simulink library "nmc"  (R2015b)
settings: Solver=ode45  SolverMode=SingleTasking  StartTime=0.0  StopTime=10.0  RelTol=1e-3
undefined symbols (not defined in the file): AnkleStance, AnkleSwing, c, c_jointstop, CtrlPar_FP_List, CtrlPar_FP_R_List, CtrlPar_LL_List, CtrlPar_St_List, CtrlPar_St_R_List, CtrlPar_Sw_List, CtrlPar_Sw_R_List, CtrlPar_theta0_List, CtrlPar_Tr_List, CtrlPar_Tr_R_List, CtrlPar_VelocityFile_List, D1G_HAT, eref, FmaxBFSH, FmaxGAS, FmaxGLU, FmaxHAB, FmaxHAD, FmaxHAM, FmaxHFL, FmaxRF, FmaxSOL, FmaxTA, FmaxVAS, init_a_tgt, init_a_tgtR, K, leg_l, LongDelay, LongLoopDelay, loptBFSH, loptGAS, loptGLU, loptHAB, loptHAD, loptHAM, loptHFL, loptRF, loptSOL, loptTA, loptVAS, lslackBFSH, lslackGAS, lslackGLU, lslackHAB, lslackHAD, lslackHAM, lslackHFL, lslackRF, lslackSOL, lslackTA, lslackVAS, magnitude, maxLoad_control_List, MeanStepsAnkle, MidDelay ... (+99)
libraries: nmc x63, simulink x31, simulink_extras x30, LopesDevelopmentLibrary x3
(part 2 of 10)

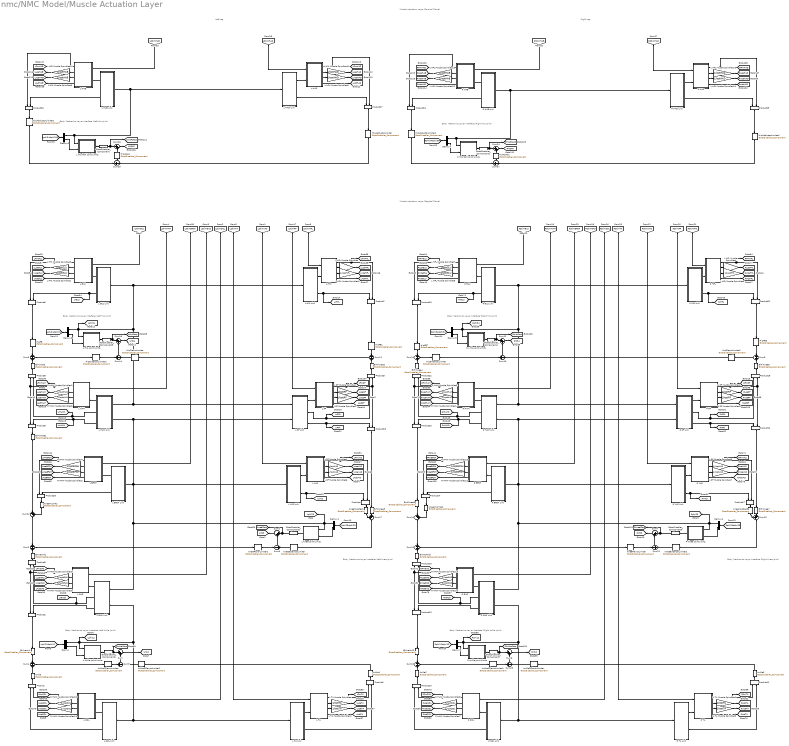
== system nmc/NMC Model/Muscle Actuation Layer ==
  note: Muscle Actuation Layer
      | (Coronal Plane)
  note: Right Leg
  note: Body Mechanics Layer
      | Interface (Right Hip Joint)
  note: Body Mechanics Layer
      | Interface (Left Hip Joint)
  note: Left Leg
  note: Body Mechanics Layer
      | Interface (Right Ankle Joint)
  note: Body Mechanics Layer
      | Interface (Right Knee Joint)
  note: Body Mechanics Layer
      | Interface (Right Hip Joint)
  note: Body Mechanics Layer
      | Interface (Left Ankle Joint)
  note: Body Mechanics Layer
      | Interface (Left Knee Joint)
  note: Body Mechanics Layer
      | Interface (Left Hip Joint)
  note: Muscle Actuation Layer
      | (Sagittal Plane)
  Ankle{,1..3} (4 alike) : nmc/GotoDisabler_Component  GotoTag=NMC_AnkleMuscles_Percentage
  AnkleDFlexorLimiter : nmc/GotoDisabler_Component  GotoTag=NMC_AnkleDFlexor_Percentage
  AnkleDFlexorLimiter1 : nmc/GotoDisabler_Component  GotoTag=NMC_AnkleDFlexor_Percentage
  AnklePFlexorLimiter : nmc/GotoDisabler_Component  GotoTag=NMC_AnklePFlexor_Percentage
  AnklePFlexorLimiter1 : nmc/GotoDisabler_Component  GotoTag=NMC_AnklePFlexor_Percentage
  BiHiKnee{,1..7} (8 alike) : nmc/GotoDisabler_Component  GotoTag=NMC_BiArticularMuscles_HK_Percentage
  BiKneAnk{,1..3} (4 alike) : nmc/GotoDisabler_Component  GotoTag=NMC_BiArticularMuscles_KA_Percentage
  Demux{,1..7} (8 alike) : Demux  Outputs=2
  GotoDisabler_Component{,1..7} (8 alike) : nmc/GotoDisabler_Component  GotoTag=DisableNMC_JointLimits
  HipAbAd : nmc/GotoDisabler_Component  GotoTag=NMC_HipAbAdMuscles_Percentage
  HipAbAd1 : nmc/GotoDisabler_Component  GotoTag=NMC_HipAbAdMuscles_Percentage
  HipAbductorLimiter1 : nmc/GotoDisabler_Component  GotoTag=NMC_HipAbductor_Percentage
  HipAbductorLimiter2 : nmc/GotoDisabler_Component  GotoTag=NMC_HipAbductor_Percentage
  HipAdductorLimiter : nmc/GotoDisabler_Component  GotoTag=NMC_HipAdductor_Percentage
  HipAdductorLimiter1 : nmc/GotoDisabler_Component  GotoTag=NMC_HipAdductor_Percentage
  HipExtensorLimiter : nmc/GotoDisabler_Component  GotoTag=NMC_HipExtensor_Percentage
  HipExtensorLimiter1 : nmc/GotoDisabler_Component  GotoTag=NMC_HipExtensor_Percentage
  HipFE{,1..3} (4 alike) : nmc/GotoDisabler_Component  GotoTag=NMC_HipFEMuscles_Percentage
  HipFlexorLimiter : nmc/GotoDisabler_Component  GotoTag=NMC_HipFlexor_Percentage
  HipFlexorLimiter1 : nmc/GotoDisabler_Component  GotoTag=NMC_HipFlexor_Percentage
  KneeExtensorLimiter : nmc/GotoDisabler_Component  GotoTag=NMC_KneeExtensor_Percentage
  KneeExtensorLimiter1 : nmc/GotoDisabler_Component  GotoTag=NMC_KneeExtensor_Percentage
  KneeFlexorLimiter : nmc/GotoDisabler_Component  GotoTag=NMC_KneeFlexor_Percentage
  KneeFlexorLimiter1 : nmc/GotoDisabler_Component  GotoTag=NMC_KneeFlexor_Percentage
  KneeMuscles{,1..3} (4 alike) : nmc/GotoDisabler_Component  GotoTag=NMC_KneeMuscles_Percentage
  L Ankle Joint Limits : Subsystem
  L BFSH : Subsystem
  L BFSH Link : Subsystem
  L GAS : Subsystem
  L GAS Link : Subsystem
  L GLU : Subsystem
  L GLU Link : Subsystem
  L HAB : Subsystem
  L HAB Link : Subsystem
  L HAD : Subsystem
  L HAD Link : Subsystem
  L HAM : Subsystem
  L HAM Link : Subsystem
  L HFL : Subsystem
  L HFL Muscle Spindles{,1,4..5} (4 alike) : Gain  Gain=1/loptHFL
  L HFL Muscle Spindles{9..10,12..13} (4 alike) : Gain  Gain=1/loptHAB
  L HFL Muscle Spindles{8,11,14..15} (4 alike) : Gain  Gain=1/loptHAD
  L HFL Muscle Spindles{2..3,6..7} (4 alike) : Gain  Gain=1/loptGLU
  L HFL Link : Subsystem
  L Hip Joint Limits : Subsystem
  L Hip Roll Joint Limits : Subsystem
  L Knee Joint Limits : Subsystem
  L RF : Subsystem
  L RF Muscle Spindles{,1..3} (4 alike) : Gain  Gain=1/loptRF
  L RF Muscle Spindles{4..7} (4 alike) : Gain  Gain=1/loptVAS
  L RF Link : Subsystem
  L SOL : Subsystem
  L SOL Link : Subsystem
  L TA : Subsystem
  L TA Muscle Spindles{,1..3} (4 alike) : Gain  Gain=1/loptTA
  L TA Link : Subsystem
  L VAS : Subsystem
  L VAS Link : Subsystem
  Product{,1..27} (28 alike) : Product  RndMeth=Zero
  R Ankle Joint Limits : Subsystem
  R BFSH : Subsystem
  R BFSH Link : Subsystem
  R GAS : Subsystem
  R GAS Link : Subsystem
  R GLU : Subsystem
  R GLU Link : Subsystem
  R HAB : Subsystem
  R HAB Link : Subsystem
  R HAD : Subsystem
  R HAD Link : Subsystem
  R HAM : Subsystem
  R HAM Muscle Spindles{1,3,6,14} (4 alike) : Gain  Gain=1/loptHAM
  R HAM Muscle Spindles{5,7,10..11} (4 alike) : Gain  Gain=1/loptSOL
  R HAM Muscle Spindles{2,4,12..13} (4 alike) : Gain  Gain=1/loptBFSH
  R HAM Muscle Spindles{8..9,15..16} (4 alike) : Gain  Gain=1/loptGAS
  R HAM Link : Subsystem
  R HFL : Subsystem
  R HFL Link : Subsystem
  R Hip Roll Joint Limits : Subsystem
  R Knee Joint Limits : Subsystem
  R L Hip Joint Limits : Subsystem
  R RF : Subsystem
  R RF Link : Subsystem
  R SOL : Subsystem
  R SOL Link : Subsystem
  R TA : Subsystem
  R TA Link : Subsystem
  R VAS : Subsystem
  R VAS Link : Subsystem
  Sum{,1,6..7,12,16,18,22,24,26} (10 alike) : Sum  Inputs=|++
  Sum{9..10,14,23,25,27} (6 alike) : Sum  Inputs=+-
  Sum{2..4,8,11,15,19..20} (8 alike) : Sum
  Sum13 : Sum  Inputs=++|
  Sum17 : Sum  Inputs=++|
  Sum21 : Sum  Inputs=-+
  Sum5 : Sum  Inputs=-+
  tag scope: LActBFSH=global, LActGAS=global, LActGLU=global, LActHAB=global, LActHAD=global, LActHAM=global, LActHFL=global, LActRF=global, LActSOL=global, LActTA=global, LActVAS=global, LAnkleStop=global, LFmBFSH=global, LFmGAS=global, LFmGLU=global, LFmHAB=global, LFmHAD=global, LFmHAM=global, LFmHFL=global, LFmRF=global, LFmSOL=global, LFmTA=global, LFmVAS=global, LHipRStop=global, LHipStop=global, LKneeStop=global, LLceBFSH=global, LLceGAS=global, LLceGLU=global, LLceHAB=global, LLceHAD=global, LLceHAM=global, LLceHFL=global, LLceRF=global, LLceSOL=global, LLceTA=global, LLceVAS=global, LM12=global, LM23=global, LM34=global, LM34R=global, LVceBFSH=global, LVceGAS=global, LVceGLU=global, LVceHAB=global, LVceHAD=global, LVceHAM=global, LVceHFL=global, LVceRF=global, LVceSOL=global, LVceTA=global, LVceVAS=global, Lphi12=global, Lphi23=global, Lphi34=global, LrGASk=global, LrGLU=global, LrHAMh=global, LrHAMk=global, LrHFL=global, LrRFh=global, LrRFk=global, LrVAS=global, RActBFSH=global, RActGAS=global, RActGLU=global, RActHAB=global, RActHAD=global, RActHAM=global, RActHFL=global, RActRF=global, RActSOL=global, RActTA=global, RActVAS=global, RAnkleStop=global, RFmBFSH=global, RFmGAS=global, RFmGLU=global, RFmHAB=global, RFmHAD=global, RFmHAM=global, RFmHFL=global, RFmRF=global, RFmSOL=global, RFmTA=global, RFmVAS=global, RHipStop=global, RHipStopR=global, RKneeStop=global, RLceBFSH=global, RLceGAS=global, RLceGLU=global, RLceHAB=global, RLceHAD=global, RLceHAM=global, RLceHFL=global, RLceRF=global, RLceSOL=global, RLceTA=global, RLceVAS=global, RM12=global, RM23=global, RM34=global, RM34R=global, RVceBFSH=global, RVceGAS=global, RVceGLU=global, RVceHAB=global, RVceHAD=global, RVceHAM=global, RVceHFL=global, RVceRF=global, RVceSOL=global, RVceTA=global, RVceVAS=global, Rphi12=global, Rphi23=global, Rphi34=global, RrGASk=global, RrGLU=global, RrHAMh=global, RrHAMk=global, RrHFL=global, RrRFh=global, RrRFk=global, RrVAS=global
  wires:
  L HFL/1(Fmtc) -> [LFmHFL], Product7/2
  [LStimHFL] -> L HFL/1(STIM)
  Product7/1 -> HipFE1/1
  Ankle3/1 -> AnkleDFlexorLimiter/1
  Ankle2/1 -> Sum20/2
  Ankle1/1 -> AnkleDFlexorLimiter1/1
  Ankle/1 -> Sum4/2
  BiKneAnk3/1 -> Sum15/2
  Product16/1 -> BiKneAnk3/1
  BiKneAnk2/1 -> Sum20/1
  BiKneAnk1/1 -> Sum2/2
  Product3/1 -> BiKneAnk1/1
  BiKneAnk/1 -> Sum4/1
  KneeMuscles3/1 -> Sum13/1
  KneeMuscles2/1 -> Sum18/2
  KneeMuscles1/1 -> Sum17/1
  KneeMuscles/1 -> Sum22/2
  Sum22/1 -> Sum2/1
  BiHiKnee7/1 -> Sum13/2
  BiHiKnee6/1 -> Sum8/2
  BiHiKnee5/1 -> Sum18/1
  BiHiKnee4/1 -> Sum19/2
  BiHiKnee3/1 -> Sum17/2
  BiHiKnee2/1 -> Sum11/2
  BiHiKnee1/1 -> Sum22/1
  Product8/1 -> BiHiKnee/1
  BiHiKnee/1 -> Sum3/2
  HipFE3/1 -> Sum8/1
  HipFE2/1 -> Sum19/1
  HipFE1/1 -> Sum11/1
  HipFE/1 -> Sum3/1
  HipAbAd1/1 -> Sum24/2
  Sum27/1 -> HipAbAd1/1
  HipAbAd/1 -> Sum26/2
  Sum25/1 -> HipAbAd/1
  AnkleDFlexorLimiter/1 -> Sum23/2
  AnkleDFlexorLimiter1/1 -> Sum9/2
  HipFlexorLimiter1/1 -> Sum10/2
  HipExtensorLimiter/1 -> Sum10/1
  HipFlexorLimiter/1 -> Sum14/2
  HipExtensorLimiter1/1 -> Sum14/1
  AnklePFlexorLimiter/1 -> Sum9/1
  AnklePFlexorLimiter1/1 -> Sum23/1
  KneeExtensorLimiter1/1 -> Sum21/2
  KneeFlexorLimiter/1 -> Sum21/1
  KneeExtensorLimiter/1 -> Sum5/2
  KneeFlexorLimiter1/1 -> Sum5/1
  Product9/1 -> BiHiKnee1/1
  HipAdductorLimiter1/1 -> Sum27/2
  HipAdductorLimiter/1 -> Sum25/2
  HipAbductorLimiter1/1 -> Sum27/1
  HipAbductorLimiter2/1 -> Sum25/1
  Product1/1 -> Ankle1/1
  Product11/1 -> Ankle3/1
  Product10/1 -> Ankle2/1
  Product/1 -> Ankle/1
  Product6/1 -> HipFE/1
  Product19/1 -> HipFE2/1
  Product21/1 -> HipFE3/1
  Product20/1 -> KneeMuscles/1
  Product14/1 -> KneeMuscles2/1
  Product17/1 -> KneeMuscles3/1
  Product4/1 -> KneeMuscles1/1
  R Ankle Joint Limits/1(M_stop [Nm]) -> GotoDisabler_Component7/1
  GotoDisabler_Component5/1 -> [LHipStop], Sum16/1
  L Hip Joint Limits/1(M_stop [Nm]) -> GotoDisabler_Component5/1
  GotoDisabler_Component4/1 -> Sum12/1, [RHipStop]
  R L Hip Joint Limits/1(M_stop [Nm]) -> GotoDisabler_Component4/1
  GotoDisabler_Component1/1 -> [RHipStopR], Sum24/1
  GotoDisabler_Component/1 -> [LHipRStop], Sum26/1
  GotoDisabler_Component2/1 -> [LKneeStop], Sum1/1
  GotoDisabler_Component3/1 -> [RKneeStop], Sum7/1
  GotoDisabler_Component6/1 -> [LAnkleStop], Sum/1
  GotoDisabler_Component7/1 -> [RAnkleStop], Sum6/1
  Sum/1 -> [LM12]
  R HAD/1(Fmtc) -> Product25/2, [RFmHAD]
  R HAD/4(A) -> [RActHAD]
  R HAD/3(Vce) -> L HFL Muscle Spindles14/1
  R HAD/2(Lce) -> L HFL Muscle Spindles15/1
  L HFL Muscle Spindles15/1 -> [RLceHAD]
  L HFL Muscle Spindles14/1 -> [RVceHAD]
  R HAB/1(Fmtc) -> Product24/1, [RFmHAB]
  L HFL Muscle Spindles13/1 -> [RLceHAB]
  L HFL Muscle Spindles12/1 -> [RVceHAB]
  R HAB/3(Vce) -> L HFL Muscle Spindles12/1
  R HAB/2(Lce) -> L HFL Muscle Spindles13/1
  R HAB/4(A) -> [RActHAB]
  L HAD/1(Fmtc) -> Product27/2, [LFmHAD]
  L HAD/4(A) -> [LActHAD]
  L HAD/3(Vce) -> L HFL Muscle Spindles8/1
  L HAD/2(Lce) -> L HFL Muscle Spindles11/1
  L HFL Muscle Spindles11/1 -> [LLceHAD]
  L HFL Muscle Spindles8/1 -> [LVceHAD]
  L HAB/1(Fmtc) -> [LFmHAB], Product26/1
  L HFL Muscle Spindles10/1 -> [LLceHAB]
  L HFL Muscle Spindles9/1 -> [LVceHAB]
  L HAB/3(Vce) -> L HFL Muscle Spindles9/1
  L HAB/2(Lce) -> L HFL Muscle Spindles10/1
  L HAB/4(A) -> [LActHAB]
  [RStimHAB] -> R HAB/1(STIM)
  R HAD Link/2(lever [m]) -> Product25/1
  R HAD Link/1(lmtu [m]) -> R HAD/2(lmtc [m])
  Product25/1 -> HipAdductorLimiter1/1
  R Hip Roll Joint Limits/1(M_stop [Nm]) -> GotoDisabler_Component1/1
  Demux7/2 -> R Hip Roll Joint Limits/2(dphi [rad/s])
  R HAB Link/2(lever [m]) -> Product24/2
  R HAB Link/1(lmtu [m]) -> R HAB/2(lmtc [m])
  Product24/1 -> HipAbductorLimiter1/1
  Demux7/1 -> R Hip Roll Joint Limits/1(phi [rad]), R HAB Link/1(phi34R [rad]), R HAD Link/1(phi34R [rad])
  [Rphi34dphi34R] -> Demux7/1
  Sum24/1 -> [RM34R]
  [RStimHAD] -> R HAD/1(STIM)
  L HAD Link/2(lever [m]) -> Product27/1
  L HAD Link/1(lmtu [m]) -> L HAD/2(lmtc [m])
  Product27/1 -> HipAdductorLimiter/1
  L Hip Roll Joint Limits/1(M_stop [Nm]) -> GotoDisabler_Component/1
  Demux6/2 -> L Hip Roll Joint Limits/2(dphi [rad/s])
  L HAB Link/2(lever [m]) -> Product26/2
  L HAB Link/1(lmtu [m]) -> L HAB/2(lmtc [m])
  Product26/1 -> HipAbductorLimiter2/1
  Demux6/1 -> L Hip Roll Joint Limits/1(phi [rad]), L HAD Link/1(phi34R [rad]), L HAB Link/1(phi34R [rad])
  [Lphi34dphi34R] -> Demux6/1
  Sum26/1 -> [LM34R]
  [LStimHAB] -> L HAB/1(STIM)
  [LStimHAD] -> L HAD/1(STIM)
  Sum11/1 -> HipFlexorLimiter/1
  L TA Muscle Spindles2/1 -> [RLceTA]
  L RF Muscle Spindles5/1 -> [RLceVAS]
  R HAM Muscle Spindles12/1 -> [RVceBFSH]
  R HAM Muscle Spindles13/1 -> [RLceBFSH]
  L RF Muscle Spindles3/1 -> [RVceRF]
  L RF Muscle Spindles1/1 -> [RLceRF]
  R HAM Muscle Spindles14/1 -> [RVceHAM]
  R HAM Muscle Spindles3/1 -> [RLceHAM]
  L HFL Muscle Spindles4/1 -> [RLceHFL]
  L TA Muscle Spindles3/1 -> [RVceTA]
  R TA/1(Fmtc) -> [RFmTA], Product11/1
  R HAM Muscle Spindles7/1 -> [RVceSOL]
  R HAM Muscle Spindles5/1 -> [RLceSOL]
  R HAM Muscle Spindles16/1 -> [RVceGAS]
  R HAM Muscle Spindles15/1 -> [RLceGAS]
  R BFSH/1(Fmtc) -> [RFmBFSH], Product14/1
  R RF/1(Fmtc) -> [RFmRF], Product12/2, Product18/2
  L RF Muscle Spindles7/1 -> [RVceVAS]
  L HFL Muscle Spindles7/1 -> [RLceGLU]
  L HFL Muscle Spindles6/1 -> [RVceGLU]
  L HFL Muscle Spindles5/1 -> [RVceHFL]
  Product23/1 -> BiHiKnee5/1
  Sum18/1 -> Sum15/1
  R BFSH/3(Vce) -> R HAM Muscle Spindles12/1
  R BFSH/2(Lce) -> R HAM Muscle Spindles13/1
  R BFSH/4(A) -> [RActBFSH]
  R BFSH Link/2(lever [m]) -> Product14/2
  R BFSH Link/1(lmtu [m]) -> R BFSH/2(lmtc [m])
  [RStimBFSH] -> R BFSH/1(STIM)
  Sum13/1 -> KneeExtensorLimiter1/1
  Product12/1 -> BiHiKnee7/1
  Product18/1 -> BiHiKnee6/1
  Sum8/1 -> HipFlexorLimiter1/1
  [RStimRF] -> R RF/1(STIM)
  R RF Link/3(lever23 [m]) -> [RrRFk], Product12/1
  R RF Link/2(lever34 [m]) -> [RrRFh], Product18/1
  R RF Link/1(lmtu [m]) -> R RF/2(lmtc [m])
  R RF/2(Lce) -> L RF Muscle Spindles1/1
  R RF/3(Vce) -> L RF Muscle Spindles3/1
  R RF/4(A) -> [RActRF]
  R HFL/3(Vce) -> L HFL Muscle Spindles5/1
  R VAS/2(Lce) -> L RF Muscle Spindles5/1
  R VAS/3(Vce) -> L RF Muscle Spindles7/1
  R TA/3(Vce) -> L TA Muscle Spindles3/1
  R SOL/3(Vce) -> R HAM Muscle Spindles7/1
  R SOL/2(Lce) -> R HAM Muscle Spindles5/1
  R GAS/2(Lce) -> R HAM Muscle Spindles15/1
  R GAS/3(Vce) -> R HAM Muscle Spindles16/1
  R HAM/3(Vce) -> R HAM Muscle Spindles14/1
  R GLU/3(Vce) -> L HFL Muscle Spindles6/1
  R GLU/2(Lce) -> L HFL Muscle Spindles7/1
  [RStimVAS] -> R VAS/1(STIM)
  R HFL Link/2(lever [m]) -> [RrHFL], Product21/1
  R HFL/4(A) -> [RActHFL]
  R HFL Link/1(lmtu [m]) -> R HFL/2(lmtc [m])
  Sum10/1 -> Sum12/2
  Demux5/2 -> R L Hip Joint Limits/2(dphi [rad/s])
  R GLU/4(A) -> [RActGLU]
  R GLU Link/2(lever [m]) -> [RrGLU], Product19/2
  R GLU Link/1(lmtu [m]) -> R GLU/2(lmtc [m])
  Product22/1 -> BiHiKnee4/1
  R HAM/4(A) -> [RActHAM]
  Sum15/1 -> KneeFlexorLimiter/1
  R VAS Link/2(lever [m]) -> Product17/1, [RrVAS]
  Sum21/1 -> Sum7/2
  R Knee Joint Limits/1(M_stop [Nm]) -> GotoDisabler_Component3/1
  Sum7/1 -> [RM23]
  R VAS/1(Fmtc) -> [RFmVAS], Product17/2
  R VAS/4(A) -> [RActVAS]
  R GAS/4(A) -> [RActGAS]
  R SOL/4(A) -> [RActSOL]
  Sum6/1 -> [RM12]
  R TA Link/2(lever [m]) -> Product11/2
  Product13/1 -> BiKneAnk2/1
  R SOL Link/2(lever [m]) -> Product10/1
  Demux5/1 -> [Rphi34], R HAM Link/1(phi34 [rad]), R RF Link/1(phi34 [rad]), R GLU Link/1(phi34 [rad]), R HFL Link/1(phi34 [rad]), R L Hip Joint Limits/1(phi [rad])
  [Rphi34dphi34] -> Demux5/1
  [Rphi23dphi23] -> Demux4/1
  [Rphi12dphi12] -> Demux3/1
  Sum20/1 -> AnklePFlexorLimiter1/1
  Sum19/1 -> HipExtensorLimiter/1
  R HAM Link/3(lever23 [m]) -> [RrHAMk], Product23/2
  R HAM Link/2(lever34 [m]) -> [RrHAMh], Product22/2
  R HAM Link/1(lmtu [m]) -> R HAM/2(lmtc [m])
  R VAS Link/1(lmtu [m]) -> R VAS/2(lmtc [m])
  R GAS Link/1(lmtu [m]) -> R GAS/2(lmtc [m])
  [RStimGAS] -> R GAS/1(STIM)
  R GAS Link/2(lever23 [m]) -> [RrGASk], Product16/2
  R GAS Link/3(lever12 [m]) -> Product13/2
  R TA Link/1(lmtc [m]) -> R TA/2(lmtc [m])
  R SOL Link/1(lmtc [m]) -> R SOL/2(lmtc [m])
  Demux4/2 -> R Knee Joint Limits/2(dphi [rad/s])
  Sum23/1 -> Sum6/2
  Demux3/2 -> R Ankle Joint Limits/2(dphi [rad/s])
  Sum12/1 -> [RM34]
  [RStimGLU] -> R GLU/1(STIM)
  R GLU/1(Fmtc) -> [RFmGLU], Product19/1
  [RStimHFL] -> R HFL/1(STIM)
  R HFL/2(Lce) -> L HFL Muscle Spindles4/1
  R HFL/1(Fmtc) -> [RFmHFL], Product21/2
  R HAM/2(Lce) -> R HAM Muscle Spindles3/1
  R HAM/1(Fmtc) -> [RFmHAM], Product22/1, Product23/1
  [RStimHAM] -> R HAM/1(STIM)
  [RStimSOL] -> R SOL/1(STIM)
  [RStimTA] -> R TA/1(STIM)
  Demux3/1 -> [Rphi12], R Ankle Joint Limits/1(phi [rad]), R GAS Link/2(phi12 [rad]), R TA Link/1(phi12 [rad]), R SOL Link/1(phi12 [rad])
  R GAS/1(Fmtc) -> [RFmGAS], Product16/1, Product13/1
  R TA/4(A) -> [RActTA]
  R TA/2(Lce) -> L TA Muscle Spindles2/1
  R SOL/1(Fmtc) -> [RFmSOL], Product10/2
  Demux4/1 -> [Rphi23], R GAS Link/1(phi23 [rad]), R BFSH Link/1(phi23 [rad]), R HAM Link/2(phi23 [rad]), R RF Link/2(phi23 [rad]), R VAS Link/1(phi23 [rad]), R Knee Joint Limits/1(phi [rad])
  L TA Muscle Spindles/1 -> [LLceTA]
  L RF Muscle Spindles4/1 -> [LLceVAS]
  R HAM Muscle Spindles2/1 -> [LVceBFSH]
  R HAM Muscle Spindles4/1 -> [LLceBFSH]
  L RF Muscle Spindles2/1 -> [LVceRF]
  L RF Muscle Spindles/1 -> [LLceRF]
  R HAM Muscle Spindles6/1 -> [LVceHAM]
  R HAM Muscle Spindles1/1 -> [LLceHAM]
  L HFL Muscle Spindles/1 -> [LLceHFL]
  L TA Muscle Spindles1/1 -> [LVceTA]
  L TA/1(Fmtc) -> [LFmTA], Product1/1
  R HAM Muscle Spindles11/1 -> [LVceSOL]
  R HAM Muscle Spindles10/1 -> [LLceSOL]
  R HAM Muscle Spindles9/1 -> [LVceGAS]
  R HAM Muscle Spindles8/1 -> [LLceGAS]
  L BFSH/1(Fmtc) -> [LFmBFSH], Product20/1
  L RF/1(Fmtc) -> [LFmRF], Product15/2, Product5/2
  L RF Muscle Spindles6/1 -> [LVceVAS]
  L HFL Muscle Spindles3/1 -> [LLceGLU]
  L HFL Muscle Spindles2/1 -> [LVceGLU]
  L HFL Muscle Spindles1/1 -> [LVceHFL]
  L BFSH/3(Vce) -> R HAM Muscle Spindles2/1
  L BFSH/2(Lce) -> R HAM Muscle Spindles4/1
  L BFSH/4(A) -> [LActBFSH]
  L BFSH Link/2(lever [m]) -> Product20/2
  L BFSH Link/1(lmtu [m]) -> L BFSH/2(lmtc [m])
  [LStimBFSH] -> L BFSH/1(STIM)
  Sum17/1 -> KneeExtensorLimiter/1
  Product15/1 -> BiHiKnee3/1
  Product5/1 -> BiHiKnee2/1
  [LStimRF] -> L RF/1(STIM)
  L RF Link/3(lever23 [m]) -> [LrRFk], Product15/1
  L RF Link/2(lever34 [m]) -> [LrRFh], Product5/1
  L RF Link/1(lmtu [m]) -> L RF/2(lmtc [m])
  L RF/2(Lce) -> L RF Muscle Spindles/1
  L RF/3(Vce) -> L RF Muscle Spindles2/1
  L RF/4(A) -> [LActRF]
  L HFL/3(Vce) -> L HFL Muscle Spindles1/1
  L VAS/2(Lce) -> L RF Muscle Spindles4/1
  L VAS/3(Vce) -> L RF Muscle Spindles6/1
  L TA/3(Vce) -> L TA Muscle Spindles1/1
  L SOL/3(Vce) -> R HAM Muscle Spindles11/1
  L SOL/2(Lce) -> R HAM Muscle Spindles10/1
  L GAS/2(Lce) -> R HAM Muscle Spindles8/1
  L GAS/3(Vce) -> R HAM Muscle Spindles9/1
  L HAM/3(Vce) -> R HAM Muscle Spindles6/1
  L GLU/3(Vce) -> L HFL Muscle Spindles2/1
  L GLU/2(Lce) -> L HFL Muscle Spindles3/1
  [LStimVAS] -> L VAS/1(STIM)
  L HFL Link/2(lever [m]) -> [LrHFL], Product7/1
  L HFL/4(A) -> [LActHFL]
  L HFL Link/1(lmtu [m]) -> L HFL/2(lmtc [m])
  Sum14/1 -> Sum16/2
  Demux2/2 -> L Hip Joint Limits/2(dphi [rad/s])
  L GLU/4(A) -> [LActGLU]
  L GLU Link/2(lever [m]) -> [LrGLU], Product6/2
  L GLU Link/1(lmtu [m]) -> L GLU/2(lmtc [m])
  L HAM/4(A) -> [LActHAM]
  Sum2/1 -> KneeFlexorLimiter1/1
  L VAS Link/2(lever [m]) -> Product4/1, [LrVAS]
  Sum5/1 -> Sum1/2
  L Knee Joint Limits/1(M_stop [Nm]) -> GotoDisabler_Component2/1
  Sum1/1 -> [LM23]
  L VAS/1(Fmtc) -> [LFmVAS], Product4/2
  L VAS/4(A) -> [LActVAS]
  L GAS/4(A) -> [LActGAS]
  L SOL/4(A) -> [LActSOL]
  L Ankle Joint Limits/1(M_stop [Nm]) -> GotoDisabler_Component6/1
  L TA Link/2(lever [m]) -> Product1/2
  Product2/1 -> BiKneAnk/1
  L SOL Link/2(lever [m]) -> Product/1
  Demux2/1 -> [Lphi34], L HAM Link/1(phi34 [rad]), L RF Link/1(phi34 [rad]), L GLU Link/1(phi34 [rad]), L HFL Link/1(phi34 [rad]), L Hip Joint Limits/1(phi [rad])
  [Lphi34dphi34] -> Demux2/1
  [Lphi23dphi23] -> Demux1/1
  [Lphi12dphi12] -> Demux/1
  Sum4/1 -> AnklePFlexorLimiter/1
  Sum3/1 -> HipExtensorLimiter1/1
  L HAM Link/3(lever23 [m]) -> [LrHAMk], Product9/2
  L HAM Link/2(lever34 [m]) -> [LrHAMh], Product8/2
  L HAM Link/1(lmtu [m]) -> L HAM/2(lmtc [m])
  L VAS Link/1(lmtu [m]) -> L VAS/2(lmtc [m])
  L GAS Link/1(lmtu [m]) -> L GAS/2(lmtc [m])
  [LStimGAS] -> L GAS/1(STIM)
  L GAS Link/2(lever23 [m]) -> [LrGASk], Product3/2
  L GAS Link/3(lever12 [m]) -> Product2/2
  L TA Link/1(lmtc [m]) -> L TA/2(lmtc [m])
  L SOL Link/1(lmtc [m]) -> L SOL/2(lmtc [m])
  Demux1/2 -> L Knee Joint Limits/2(dphi [rad/s])
  Sum9/1 -> Sum/2
  Demux/2 -> L Ankle Joint Limits/2(dphi [rad/s])
  Sum16/1 -> [LM34]
  [LStimGLU] -> L GLU/1(STIM)
  L GLU/1(Fmtc) -> [LFmGLU], Product6/1
  L HFL/2(Lce) -> L HFL Muscle Spindles/1
  L HAM/2(Lce) -> R HAM Muscle Spindles1/1
  L HAM/1(Fmtc) -> [LFmHAM], Product8/1, Product9/1
  [LStimHAM] -> L HAM/1(STIM)
  [LStimSOL] -> L SOL/1(STIM)
  [LStimTA] -> L TA/1(STIM)
  Demux/1 -> [Lphi12], L Ankle Joint Limits/1(phi [rad]), L GAS Link/2(phi12 [rad]), L TA Link/1(phi12 [rad]), L SOL Link/1(phi12 [rad])
  L GAS/1(Fmtc) -> [LFmGAS], Product3/1, Product2/1
  L TA/4(A) -> [LActTA]
  L TA/2(Lce) -> L TA Muscle Spindles/1
  L SOL/1(Fmtc) -> [LFmSOL], Product/2
  Demux1/1 -> [Lphi23], L GAS Link/1(phi23 [rad]), L BFSH Link/1(phi23 [rad]), L HAM Link/2(phi23 [rad]), L RF Link/2(phi23 [rad]), L VAS Link/1(phi23 [rad]), L Knee Joint Limits/1(phi [rad])

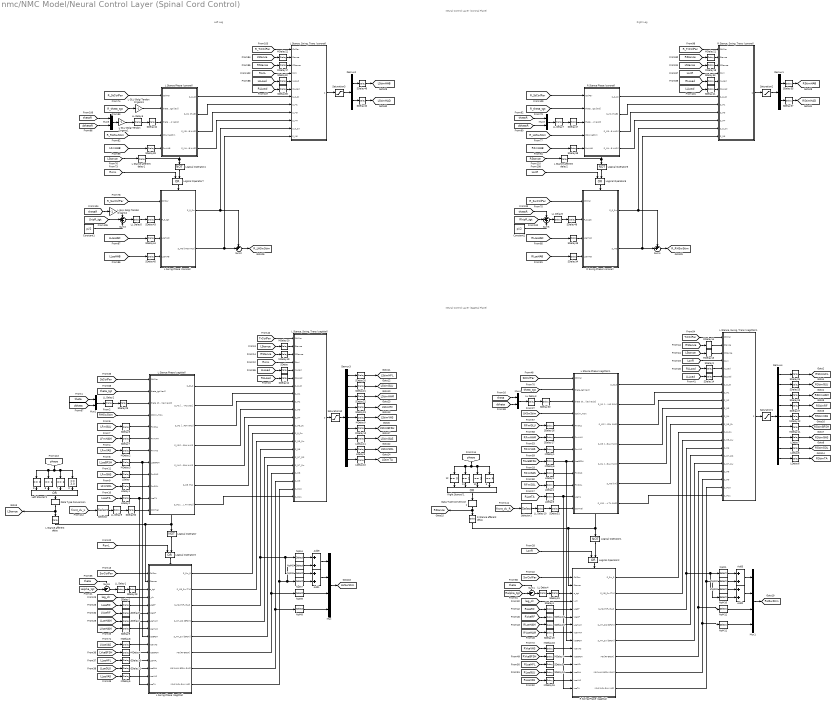
== system nmc/NMC Model/Neural Control Layer (Spinal Cord Control) ==
  note: Neural Control Layer
      | (Sagittal Plane)
  note: Neural Control Layer
      | (Coronal Plane)
  note: Right Leg
  note: Left Leg
  " 2" : simulink/Logic and Bit Operations/Compare To Constant  relop===  const=3.0  OutDataTypeStr=boolean
  " 3" : simulink/Logic and Bit Operations/Compare To Constant  relop===  const=4  OutDataTypeStr=boolean
  10 : simulink/Logic and Bit Operations/Compare To Constant  relop===  const=3  OutDataTypeStr=boolean
  11 : simulink/Logic and Bit Operations/Compare To Constant  relop===  const=1  OutDataTypeStr=boolean
  12 : simulink/Logic and Bit Operations/Compare To Constant  relop===  const=0  OutDataTypeStr=boolean
  7 : simulink/Logic and Bit Operations/Compare To Constant  relop===  const=2  OutDataTypeStr=boolean
  8 : simulink/Logic and Bit Operations/Compare To Constant  relop===  const=1  OutDataTypeStr=boolean
  9 : simulink/Logic and Bit Operations/Compare To Constant  relop===  const=0  OutDataTypeStr=boolean
  Add{1..3,9} (4 alike) : Sum  Inputs=2
  Constant1 : Constant  Value=pi/2
  Constant2 : Constant  Value=pi/2
  Data Type Conversion : DataTypeConversion
  Data Type Conversion1 : DataTypeConversion
  Demux1 : Demux  Outputs=2
  Demux2 : Demux  Outputs=2
  Demux3 : Demux  Outputs=9
  Demux4 : Demux  Outputs=9
  L GLU Golgi Tendon Organs1 : Gain  Gain=-1
  L GLU Golgi Tendon Organs2 : Gain  Gain=-1
  L GLU Golgi Tendon Organs3 : Gain  Gain=-1
  L Stance afferent delay : TransportDelay  DelayTime=MidDelay
  L Stance afferent delay1 : TransportDelay  DelayTime=MidDelay
  L Stance afferent delay2 : TransportDelay  DelayTime=MidDelay
  L Stance Phase (coronal) : Subsystem  TreatAsAtomicUnit=on
  L Stance Phase (sagittal) : Subsystem  TreatAsAtomicUnit=on
  L Stance Phase (sagittal)1 : Subsystem  TreatAsAtomicUnit=on
  "L Stance, Swing, Trans (coronal)" : Subsystem  TreatAsAtomicUnit=on
  "L Stance, Swing, Trans (sagittal)" : Subsystem
  "L Stance, Swing, Trans (sagittal)1" : Subsystem
  L Swing Phase (coronal) : Subsystem  TreatAsAtomicUnit=on
  L Swing Phase (sagittal) : Subsystem  TreatAsAtomicUnit=on
  LDelay{,1,3..4} (4 alike) : TransportDelay  DelayTime=LongDelay
  LDelay10 : TransportDelay  DelayTime=LongDelay  InitialOutput=St_PreSTA
  LDelay11 : TransportDelay  DelayTime=LongDelay  InitialOutput=St_PreSGAS
  LDelay2 : TransportDelay  DelayTime=LongDelay  InitialOutput=1
  LDelay5 : TransportDelay  DelayTime=LongDelay  InitialOutput=1
  LDelay6 : TransportDelay  DelayTime=LongDelay  InitialOutput=Sw_PreSTA
  LDelay7 : TransportDelay  DelayTime=LongDelay  InitialOutput=Sw_PreSGAS
  LDelay8 : TransportDelay  DelayTime=LongDelay  InitialOutput=Sw_PreSSOL
  LDelay9 : TransportDelay  DelayTime=LongDelay  InitialOutput=St_PreSSOL
  LL Delay1 : TransportDelay  DelayTime=LongLoopDelay/2  InitialOutput=init_a_tgt
  LL Delay{2..3,6..7,9..10} (6 alike) : TransportDelay  DelayTime=LongLoopDelay/2
  LL Delay4 : TransportDelay  DelayTime=LongLoopDelay/2  InitialOutput=init_a_tgt
  LL Delay5 : TransportDelay  DelayTime=LongLoopDelay/2  InitialOutput=init_a_tgtR
  LL Delay8 : TransportDelay  DelayTime=LongLoopDelay/2  InitialOutput=init_a_tgtR
  Left Stance?2 : Logic  Operator=OR  Inputs=4  AllPortsSameDT=off
  Logical Operator{,1,4..5} (4 alike) : Logic  Operator=NOT  AllPortsSameDT=off  OutDataTypeStr=boolean
  Logical Operator{2..3,6..7} (4 alike) : Logic  Operator=OR  AllPortsSameDT=off  OutDataTypeStr=boolean
  MDelay{1..2,4,7..8,13..14,16..22} (14 alike) : TransportDelay  DelayTime=MidDelay
  MDelay10 : TransportDelay  DelayTime=MidDelay  InitialOutput=St_PreSBFSH
  MDelay11 : TransportDelay  DelayTime=MidDelay  InitialOutput=Sw_PreSBFSH
  MDelay12 : TransportDelay  DelayTime=MidDelay  InitialOutput=Sw_PreSVAS
  MDelay{3,5..6,15} (4 alike) : TransportDelay  DelayTime=MidDelay  InitialOutput=1
  MDelay9 : TransportDelay  DelayTime=MidDelay  InitialOutput=St_PreSVAS
  Mux : Mux
  Mux1 : Mux
  Mux{2..5} (4 alike) : Mux  Inputs=2
  R Stance afferent delay : TransportDelay  DelayTime=MidDelay
  R Stance Phase (coronal) : Subsystem  TreatAsAtomicUnit=on
  "R Stance, Swing, Trans (coronal)" : Subsystem  TreatAsAtomicUnit=on
  R Swing Phase (coronal) : Subsystem  TreatAsAtomicUnit=on
  R Swing Phase (sagittal) : Subsystem  TreatAsAtomicUnit=on
  Right Stance?1 : Logic  Operator=OR  Inputs=4  AllPortsSameDT=off
  SDelay{,3,6..9,12,14,16..19,29..30,32..33,36,38..39,41..42,47,50..51} (24 alike) : TransportDelay  DelayTime=ShortDelay
  SDelay{1..2,4..5,10..11,13,15,34,44..45,49} (12 alike) : TransportDelay  DelayTime=ShortDelay  InitialOutput=1
  SDelay20 : TransportDelay  DelayTime=ShortDelay  InitialOutput=St_PreSHFL
  SDelay21 : TransportDelay  DelayTime=ShortDelay  InitialOutput=St_PreSGLU
  SDelay22 : TransportDelay  DelayTime=ShortDelay  InitialOutput=St_PreSHAM
  SDelay23 : TransportDelay  DelayTime=ShortDelay  InitialOutput=St_PreSRF
  SDelay24 : TransportDelay  DelayTime=ShortDelay  InitialOutput=Sw_PreSHFL
  SDelay25 : TransportDelay  DelayTime=ShortDelay  InitialOutput=Sw_PreSGLU
  SDelay26 : TransportDelay  DelayTime=ShortDelay  InitialOutput=Sw_PreSHAM
  SDelay27 : TransportDelay  DelayTime=ShortDelay  InitialOutput=Sw_PreSRF
  SDelay28 : TransportDelay  DelayTime=ShortDelay  InitialOutput=init_a_tgt
  SDelay31 : TransportDelay  DelayTime=ShortDelay  InitialOutput=init_a_tgt
  SDelay35 : TransportDelay  DelayTime=ShortDelay  InitialOutput=Sw_PreS_HAB
  SDelay37 : TransportDelay  DelayTime=ShortDelay  InitialOutput=Sw_PreS_HAD
  SDelay40 : TransportDelay  DelayTime=ShortDelay  InitialOutput=St_PreS_HAD
  SDelay43 : TransportDelay  DelayTime=ShortDelay  InitialOutput=init_a_tgtR
  SDelay46 : TransportDelay  DelayTime=ShortDelay  InitialOutput=St_PreS_HAB
  SDelay48 : TransportDelay  DelayTime=ShortDelay  InitialOutput=init_a_tgtR
  Saturation{1..3,10} (4 alike) : Saturate  UpperLimit=1  LowerLimit=0.01  ZeroCross=off
  Selector : Selector  InputPortWidth=2  IndexOptions=Index vector (dialog)  Indices=[2]  OutputSizes=1
  Selector1 : Selector  InputPortWidth=2  IndexOptions=Index vector (dialog)  Indices=[2]  OutputSizes=1
  Sum1 : Sum  Inputs=-+|
  Sum2 : Sum  Inputs=++|
  Sum3 : Sum  Inputs=--+
  Sum4 : Sum  Inputs=++|
  Sum5 : Sum  Inputs=--+
  Sum6 : Sum  Inputs=-+|
  hipM{1,4,9,12} (4 alike) : Selector  InputPortWidth=2  IndexOptions=Index vector (dialog)  Indices=1  OutputSizes=1
  hipM10 : Selector  InputPortWidth=3  IndexOptions=Index vector (dialog)  Indices=2  OutputSizes=1
  hipM{2,5,8,11} (4 alike) : Selector  InputPortWidth=3  IndexOptions=Index vector (dialog)  Indices=1  OutputSizes=1
  hipM3 : Selector  InputPortWidth=2  IndexOptions=Index vector (dialog)  Indices=2  OutputSizes=1
  hipM6 : Selector  InputPortWidth=2  IndexOptions=Index vector (dialog)  Indices=2  OutputSizes=1
  hipM7 : Selector  InputPortWidth=3  IndexOptions=Index vector (dialog)  Indices=2  OutputSizes=1
  tag scope: LHSwStim=global, LStance=global, LStimBFSH=global, LStimGAS=global, LStimGLU=global, LStimHAB=global, LStimHAD=global, LStimHAM=global, LStimHFL=global, LStimRF=global, LStimSOL=global, LStimTA=global, LStimVAS=global, RHSwStim=global, RStance=global, RStimBFSH=global, RStimGAS=global, RStimGLU=global, RStimHAB=global, RStimHAD=global, RStimHAM=global, RStimHFL=global, RStimRF=global, RStimSOL=global, RStimTA=global, RStimVAS=global, R_LHSwStim=global, R_RHSwStim=global
  wires:
  Data Type Conversion1/1 -> R Stance afferent delay/1, [RStance]
  Data Type Conversion/1 -> L Stance afferent delay/1, [LStance]
  [phase] -> 11/1, 12/1, 10/1, " 3"/1
  " 3"/1 -> Right Stance?1/4
  10/1 -> Right Stance?1/3
  11/1 -> Right Stance?1/2
  12/1 -> Right Stance?1/1
  [phase] -> 8/1, 9/1, 7/1, " 2"/1
  " 2"/1 -> Left Stance?2/4
  7/1 -> Left Stance?2/3
  8/1 -> Left Stance?2/2
  9/1 -> Left Stance?2/1
  [LLLoad] -> SDelay/1
  Left Stance?2/1 -> Data Type Conversion/1
  [StCtrlPar] -> L Stance Phase (sagittal)/1(CtrlPar)
  [RHSwStim] -> L Stance Phase (sagittal)/4(CStim_HSw)
  [LFmGLU] -> SDelay6/1
  SDelay6/1 -> L Stance Phase (sagittal)/5(FmGLU)
  [LFmHAM] -> SDelay7/1
  SDelay7/1 -> L Stance Phase (sagittal)/6(FmHAM)
  [LFmVAS] -> MDelay2/1
  MDelay2/1 -> L Stance Phase (sagittal)/7(FmVAS)
  [LLceBFSH] -> MDelay3/1
  MDelay3/1 -> L Swing Phase (sagittal)/9(lceBFSH), L Stance Phase (sagittal)/8(LceBFSH)
  [LFmGAS] -> LDelay/1
  LDelay/1 -> L Stance Phase (sagittal)/9(FmGAS)
  [LFmSOL] -> LDelay1/1
  LDelay1/1 -> L Stance Phase (sagittal)/10(FmSOL)
  [LLceTA] -> LDelay2/1
  LDelay2/1 -> L Swing Phase (sagittal)/15(LceTA), L Stance Phase (sagittal)/11(LceTA)
  [SwCtrlPar] -> L Swing Phase (sagittal)/1(CtrlPar)
  L Stance afferent delay/1 -> L Stance Phase (sagittal)/Enable, Logical Operator/1, L Swing Phase (sagittal)/2(Stance)
  Logical Operator/1 -> Logical Operator3/2
  Logical Operator3/1 -> L Swing Phase (sagittal)/Enable
  [RonL] -> Logical Operator3/1
  [leg_clr] -> L Swing Phase (sagittal)/4(l_clr)
  [LLceRF] -> SDelay1/1
  SDelay1/1 -> L Swing Phase (sagittal)/5(LceRF)
  [LLceHAM] -> SDelay2/1
  SDelay2/1 -> L Swing Phase (sagittal)/7(LceHAM)
  [LVceRF] -> SDelay8/1
  SDelay8/1 -> L Swing Phase (sagittal)/6(VceRF)
  [LVceHAM] -> SDelay9/1
  SDelay9/1 -> L Swing Phase (sagittal)/8(VceHAM)
  [LVceBFSH] -> MDelay4/1
  MDelay4/1 -> L Swing Phase (sagittal)/11(VceBFSH)
  SDelay10/1 -> L Swing Phase (sagittal)/12(LceHFL)
  SDelay11/1 -> L Swing Phase (sagittal)/13(LceGLU)
  MDelay5/1 -> L Swing Phase (sagittal)/14(LceVAS)
  [TrCtrlPar] -> "L Stance, Swing, Trans (sagittal)"/1(CtrlPar)
  [RLLoad] -> SDelay12/1
  Demux3/1 -> SDelay20/1
  Demux3/2 -> SDelay21/1
  Demux3/3 -> SDelay22/1
  Saturation10/1 -> Demux3/1
  Demux3/7 -> LDelay11/1
  Demux3/8 -> LDelay9/1
  Demux3/9 -> LDelay10/1
  Demux3/4 -> SDelay23/1
  Demux3/5 -> MDelay9/1
  Demux3/6 -> MDelay10/1
  "L Stance, Swing, Trans (sagittal)"/1(S) -> Saturation10/1
  [RonL] -> "L Stance, Swing, Trans (sagittal)"/4(ConI)
  [LStance] -> MDelay20/1
  [RStance] -> MDelay19/1
  Right Stance?1/1 -> Data Type Conversion1/1
  [StCtrlPar] -> L Stance Phase (sagittal)1/1(CtrlPar)
  [RLLoad] -> SDelay3/1
  [LHSwStim] -> L Stance Phase (sagittal)1/4(CStim_HSw)
  [RFmGLU] -> SDelay16/1
  SDelay16/1 -> L Stance Phase (sagittal)1/5(FmGLU)
  [RFmHAM] -> SDelay17/1
  SDelay17/1 -> L Stance Phase (sagittal)1/6(FmHAM)
  [RFmVAS] -> MDelay1/1
  MDelay1/1 -> L Stance Phase (sagittal)1/7(FmVAS)
  [RLceBFSH] -> MDelay6/1
  MDelay6/1 -> R Swing Phase (sagittal)/9(lceBFSH), L Stance Phase (sagittal)1/8(LceBFSH)
  [RFmGAS] -> LDelay3/1
  LDelay3/1 -> L Stance Phase (sagittal)1/9(FmGAS)
  [RFmSOL] -> LDelay4/1
  LDelay4/1 -> L Stance Phase (sagittal)1/10(FmSOL)
  [RLceTA] -> LDelay5/1
  LDelay5/1 -> R Swing Phase (sagittal)/15(LceTA), L Stance Phase (sagittal)1/11(LceTA)
  [SwCtrlPar] -> R Swing Phase (sagittal)/1(CtrlPar)
  R Stance afferent delay/1 -> R Swing Phase (sagittal)/2(Stance), Logical Operator1/1, L Stance Phase (sagittal)1/Enable
  Logical Operator1/1 -> Logical Operator2/2
  Logical Operator2/1 -> R Swing Phase (sagittal)/Enable
  [LonR] -> Logical Operator2/1
  [leg_clr] -> R Swing Phase (sagittal)/4(l_clr)
  [RLceRF] -> SDelay4/1
  SDelay4/1 -> R Swing Phase (sagittal)/5(LceRF)
  [RLceHAM] -> SDelay15/1
  SDelay15/1 -> R Swing Phase (sagittal)/7(LceHAM)
  [RVceRF] -> SDelay18/1
  SDelay18/1 -> R Swing Phase (sagittal)/6(VceRF)
  [RVceHAM] -> SDelay19/1
  SDelay19/1 -> R Swing Phase (sagittal)/8(VceHAM)
  [RVceBFSH] -> MDelay7/1
  MDelay7/1 -> R Swing Phase (sagittal)/11(VceBFSH)
  SDelay5/1 -> R Swing Phase (sagittal)/12(LceHFL)
  SDelay13/1 -> R Swing Phase (sagittal)/13(LceGLU)
  MDelay15/1 -> R Swing Phase (sagittal)/14(LceVAS)
  [TrCtrlPar] -> "L Stance, Swing, Trans (sagittal)1"/1(CtrlPar)
  SDelay14/1 -> "L Stance, Swing, Trans (sagittal)1"/6(CLLoad)
  [LLLoad] -> SDelay14/1
  Saturation1/1 -> Demux4/1
  [LonR] -> "L Stance, Swing, Trans (sagittal)1"/4(ConI)
  [RStance] -> MDelay14/1
  [LStance] -> MDelay13/1
  SDelay12/1 -> "L Stance, Swing, Trans (sagittal)"/6(CLLoad)
  SDelay20/1 -> [LStimHFL]
  SDelay21/1 -> [LStimGLU]
  SDelay22/1 -> [LStimHAM]
  SDelay23/1 -> [LStimRF]
  MDelay9/1 -> [LStimVAS]
  MDelay10/1 -> [LStimBFSH]
  LDelay11/1 -> [LStimGAS]
  LDelay9/1 -> [LStimSOL]
  LDelay10/1 -> [LStimTA]
  Demux4/1 -> SDelay24/1
  Demux4/2 -> SDelay25/1
  Demux4/3 -> SDelay26/1
  Demux4/7 -> LDelay7/1
  Demux4/8 -> LDelay8/1
  Demux4/9 -> LDelay6/1
  Demux4/4 -> SDelay27/1
  Demux4/5 -> MDelay12/1
  Demux4/6 -> MDelay11/1
  SDelay24/1 -> [RStimHFL]
  SDelay25/1 -> [RStimGLU]
  SDelay26/1 -> [RStimHAM]
  SDelay27/1 -> [RStimRF]
  MDelay12/1 -> [RStimVAS]
  MDelay11/1 -> [RStimBFSH]
  LDelay7/1 -> [RStimGAS]
  LDelay8/1 -> [RStimSOL]
  LDelay6/1 -> [RStimTA]
  [Lalpha_tgt] -> Sum6/2
  [theta] -> Sum6/1
  [Ralpha_tgt] -> Sum1/2
  [theta] -> Sum1/1
  MDelay20/1 -> "L Stance, Swing, Trans (sagittal)"/2(Stance)
  MDelay19/1 -> "L Stance, Swing, Trans (sagittal)"/3(CStance)
  MDelay14/1 -> "L Stance, Swing, Trans (sagittal)1"/2(Stance)
  MDelay13/1 -> "L Stance, Swing, Trans (sagittal)1"/3(CStance)
  [LLceHFL] -> SDelay10/1
  [LLceGLU] -> SDelay11/1
  [LLceVAS] -> MDelay5/1
  [RLceHFL] -> SDelay5/1
  [RLceGLU] -> SDelay13/1
  [RLceVAS] -> MDelay15/1
  LL Delay1/1 -> SDelay28/1
  Sum6/1 -> LL Delay1/1
  SDelay28/1 -> L Swing Phase (sagittal)/3(a_tgt)
  L Stance Phase (sagittal)/1(S_St_0) -> "L Stance, Swing, Trans (sagittal)"/7(S_0_St)
  L Swing Phase (sagittal)/1(S_Sw_0) -> "L Stance, Swing, Trans (sagittal)"/13(S_0_Sw)
  L Stance Phase (sagittal)1/1(S_St_0) -> "L Stance, Swing, Trans (sagittal)1"/7(S_0_St)
  L Stance Phase (sagittal)/2(S_M1 [GLU VAS SOL]) -> "L Stance, Swing, Trans (sagittal)"/8(S_M1)
  L Stance Phase (sagittal)/3(S_M2 [HAM VAS BFSH GAS]) -> "L Stance, Swing, Trans (sagittal)"/9(S_M2)
  L Stance Phase (sagittal)/6(S_M5 [TA]) -> "L Stance, Swing, Trans (sagittal)"/12(S_M5_St)
  L Stance Phase (sagittal)1/2(S_M1 [GLU VAS SOL]) -> "L Stance, Swing, Trans (sagittal)1"/8(S_M1)
  L Stance Phase (sagittal)1/3(S_M2 [HAM VAS BFSH GAS]) -> "L Stance, Swing, Trans (sagittal)1"/9(S_M2)
  L Stance Phase (sagittal)1/6(S_M5 [TA]) -> "L Stance, Swing, Trans (sagittal)1"/12(S_M5_St)
  [theta] -> Mux2/1
  [dtheta] -> Mux2/2
  [theta_tgt] -> L Stance Phase (sagittal)/2(theta_tgt [rad])
  SDelay/1 -> "L Stance, Swing, Trans (sagittal)"/5(ILLoad)
  [theta] -> Mux4/1
  [dtheta] -> Mux4/2
  [theta_tgt] -> L Stance Phase (sagittal)1/2(theta_tgt [rad])
  L Stance Phase (sagittal)/4(S_M3 [HFL GLU HAM]) -> "L Stance, Swing, Trans (sagittal)"/10(S_M3)
  L Stance Phase (sagittal)1/4(S_M3 [HFL GLU HAM]) -> "L Stance, Swing, Trans (sagittal)1"/10(S_M3)
  SDelay3/1 -> "L Stance, Swing, Trans (sagittal)1"/5(ILLoad)
  LL Delay2/1 -> SDelay29/1
  Mux2/1 -> LL Delay2/1
  SDelay29/1 -> L Stance Phase (sagittal)/3(theta dtheta [rad rad/s])
  LL Delay3/1 -> SDelay30/1
  Mux4/1 -> LL Delay3/1
  SDelay30/1 -> L Stance Phase (sagittal)1/3(theta dtheta [rad rad/s])
  L Stance Phase (sagittal)1/5(S_M4 [HFL GLU HAM]) -> "L Stance, Swing, Trans (sagittal)1"/11(S_M4)
  L Stance Phase (sagittal)/5(S_M4 [HFL GLU HAM]) -> "L Stance, Swing, Trans (sagittal)"/11(S_M4)
  L Swing Phase (sagittal)/2(S_M5_Sw [TA]) -> "L Stance, Swing, Trans (sagittal)"/14(S_M5_Sw)
  L Swing Phase (sagittal)/3(S_M6 [HFL GLU]) -> "L Stance, Swing, Trans (sagittal)"/15(S_M6), hipM6/1, hipM4/1
  L Swing Phase (sagittal)/4(S_M7_DS [BFSH]) -> "L Stance, Swing, Trans (sagittal)"/16(S_M7_DS)
  L Swing Phase (sagittal)/5(S_M7_Sw [BFSH]) -> "L Stance, Swing, Trans (sagittal)"/17(S_M7_Sw)
  L Swing Phase (sagittal)/6(M8 [RF BFSH]) -> "L Stance, Swing, Trans (sagittal)"/18(S_M8), hipM9/1
  L Swing Phase (sagittal)/7(M9 [HAM BFSH GAS]) -> "L Stance, Swing, Trans (sagittal)"/19(S_M9), hipM8/1
  L Swing Phase (sagittal)/8(M10 [HFL GLU VAS]) -> "L Stance, Swing, Trans (sagittal)"/20(S_M10), hipM5/1, hipM7/1
  Mux/1 -> [LHSwStim]
  hipM4/1 -> Add9/1
  hipM5/1 -> Add9/2
  Add9/1 -> Mux/1
  hipM6/1 -> Add1/1
  hipM7/1 -> Add1/2
  Add1/1 -> Mux/2
  hipM9/1 -> Mux/3
  hipM8/1 -> Mux/4
  "L Stance, Swing, Trans (sagittal)1"/1(S) -> Saturation1/1
  R Swing Phase (sagittal)/1(S_Sw_0) -> "L Stance, Swing, Trans (sagittal)1"/13(S_0_Sw)
  R Swing Phase (sagittal)/2(S_M5_Sw [TA]) -> "L Stance, Swing, Trans (sagittal)1"/14(S_M5_Sw)
  R Swing Phase (sagittal)/3(S_M6 [HFL GLU]) -> "L Stance, Swing, Trans (sagittal)1"/15(S_M6), hipM3/1, hipM1/1
  R Swing Phase (sagittal)/4(S_M7_DS [BFSH]) -> "L Stance, Swing, Trans (sagittal)1"/16(S_M7_DS)
  R Swing Phase (sagittal)/5(S_M7_Sw [BFSH]) -> "L Stance, Swing, Trans (sagittal)1"/17(S_M7_Sw)
  R Swing Phase (sagittal)/6(M8 [RF BFSH]) -> "L Stance, Swing, Trans (sagittal)1"/18(S_M8), hipM12/1
  R Swing Phase (sagittal)/7(M9 [HAM BFSH GAS]) -> "L Stance, Swing, Trans (sagittal)1"/19(S_M9), hipM11/1
  R Swing Phase (sagittal)/8(M10 [HFL GLU VAS]) -> "L Stance, Swing, Trans (sagittal)1"/20(S_M10), hipM2/1, hipM10/1
  Mux1/1 -> [RHSwStim]
  hipM1/1 -> Add3/1
  hipM2/1 -> Add3/2
  Add3/1 -> Mux1/1
  hipM3/1 -> Add2/1
  hipM10/1 -> Add2/2
  Add2/1 -> Mux1/2
  hipM12/1 -> Mux1/3
  hipM11/1 -> Mux1/4
  LL Delay4/1 -> SDelay31/1
  Sum1/1 -> LL Delay4/1
  SDelay31/1 -> R Swing Phase (sagittal)/3(a_tgt)
  [LVceVAS] -> MDelay8/1
  MDelay8/1 -> L Swing Phase (sagittal)/10(VceVAS)
  [RVceVAS] -> MDelay16/1
  MDelay16/1 -> R Swing Phase (sagittal)/10(VceVAS)
  Logical Operator5/1 -> Logical Operator6/2
  Logical Operator6/1 -> R Swing Phase (coronal)/Enable
  [LonR] -> Logical Operator6/1
  [RStance] -> L Stance afferent delay2/1
  L Stance afferent delay2/1 -> Logical Operator5/1, R Stance Phase (coronal)/Enable
  [R_StCtrlPar] -> R Stance Phase (coronal)/1(CtrlPar)
  [R_LHSwStim] -> R Stance Phase (coronal)/4(CSwingStim)
  [R_SwCtrlPar] -> R Swing Phase (coronal)/1(CtrlPar)
  [R_TrCtrlPar] -> "R Stance, Swing, Trans (coronal)"/1(CtrlPar)
  [LonR] -> "R Stance, Swing, Trans (coronal)"/4(ConI)
  [LLLoad] -> SDelay41/1
  SDelay41/1 -> "R Stance, Swing, Trans (coronal)"/6(CLLoad)
  Saturation2/1 -> Demux1/1
  Demux1/2 -> SDelay37/1
  Demux1/1 -> SDelay35/1
  [RLLoad] -> SDelay33/1
  [R_theta_tgt] -> R Stance Phase (coronal)/2(theta_tgt [rad])
  R Swing Phase (coronal)/2(S_M6) -> Sum4/2, "R Stance, Swing, Trans (coronal)"/12(S_M6)
  Sum4/1 -> [R_RHSwStim]
  SDelay33/1 -> "R Stance, Swing, Trans (coronal)"/5(ILLoad)
  R Stance Phase (coronal)/1(S_0_St) -> "R Stance, Swing, Trans (coronal)"/7(S_0_St)
  R Stance Phase (coronal)/3(S_M3 [HAB HAD]) -> "R Stance, Swing, Trans (coronal)"/9(S_M3)
  R Stance Phase (coronal)/4(S_M4 [HAB HAD]) -> "R Stance, Swing, Trans (coronal)"/10(S_M4)
  R Swing Phase (coronal)/1(S_0_Sw) -> Sum4/1, "R Stance, Swing, Trans (coronal)"/11(S_0_Sw)
  [RLceHAD] -> SDelay49/1
  [RLceHAB] -> SDelay34/1
  [RhipR_tgt] -> Sum5/2
  Constant2/1 -> Sum5/3
  [thetaR] -> Sum5/1
  LL Delay7/1 -> SDelay47/1
  SDelay47/1 -> R Stance Phase (coronal)/3(theta dtheta [rad rad/s])
  Mux3/1 -> LL Delay7/1
  LL Delay8/1 -> SDelay48/1
  SDelay48/1 -> R Swing Phase (coronal)/2(R_a_tgt)
  Sum5/1 -> LL Delay8/1
  SDelay49/1 -> R Swing Phase (coronal)/3(LceHAD)
  SDelay34/1 -> R Swing Phase (coronal)/4(LceHAB)
  MDelay21/1 -> "R Stance, Swing, Trans (coronal)"/2(Stance)
  [RStance] -> MDelay21/1
  [LStance] -> MDelay18/1
  MDelay18/1 -> "R Stance, Swing, Trans (coronal)"/3(CStance)
  "R Stance, Swing, Trans (coronal)"/1(S) -> Saturation2/1
  [thetaR] -> Mux3/1
  [dthetaR] -> Mux3/2
  R Stance Phase (coronal)/2(S_M1 [HAB]) -> "R Stance, Swing, Trans (coronal)"/8(S_M1)
  [RFmHAB] -> SDelay38/1
  SDelay38/1 -> R Stance Phase (coronal)/5(FmHAB)
  Logical Operator4/1 -> Logical Operator7/2
  Logical Operator7/1 -> L Swing Phase (coronal)/Enable
  [RonL] -> Logical Operator7/1
  [LStance] -> L Stance afferent delay1/1
  L Stance afferent delay1/1 -> Logical Operator4/1, L Stance Phase (coronal)/Enable
  L GLU Golgi Tendon Organs3/1 -> L Stance Phase (coronal)/2(theta_tgt [rad])
  [R_StCtrlPar] -> L Stance Phase (coronal)/1(CtrlPar)
  [R_RHSwStim] -> L Stance Phase (coronal)/4(CSwingStim)
  [R_SwCtrlPar] -> L Swing Phase (coronal)/1(CtrlPar)
  [R_TrCtrlPar] -> "L Stance, Swing, Trans (coronal)"/1(CtrlPar)
  [RonL] -> "L Stance, Swing, Trans (coronal)"/4(ConI)
  [LStance] -> MDelay22/1
  [RStance] -> MDelay17/1
  [RLLoad] -> SDelay36/1
  SDelay36/1 -> "L Stance, Swing, Trans (coronal)"/6(CLLoad)
  Saturation3/1 -> Demux2/1
  Demux2/2 -> SDelay40/1
  Demux2/1 -> SDelay46/1
  [LLLoad] -> SDelay32/1
  [R_theta_tgt] -> L GLU Golgi Tendon Organs3/1
  Mux5/1 -> L GLU Golgi Tendon Organs1/1
  L Swing Phase (coronal)/2(S_M6 [HAB HAD]) -> Sum2/2, "L Stance, Swing, Trans (coronal)"/12(S_M6)
  Sum2/1 -> [R_LHSwStim]
  SDelay32/1 -> "L Stance, Swing, Trans (coronal)"/5(ILLoad)
  L Stance Phase (coronal)/1(S_0_St) -> "L Stance, Swing, Trans (coronal)"/7(S_0_St)
  L Stance Phase (coronal)/3(S_M3 [HAB HAD]) -> "L Stance, Swing, Trans (coronal)"/9(S_M3)
  L Stance Phase (coronal)/4(S_M4 [HAB HAD]) -> "L Stance, Swing, Trans (coronal)"/10(S_M4)
  L Swing Phase (coronal)/1(S_0_Sw) -> "L Stance, Swing, Trans (coronal)"/11(S_0_Sw), Sum2/1
  [LLceHAD] -> SDelay44/1
  [LLceHAB] -> SDelay45/1
  Constant1/1 -> Sum3/3
  LL Delay6/1 -> SDelay42/1
  SDelay42/1 -> L Stance Phase (coronal)/3(theta dtheta [rad rad/s])
  L GLU Golgi Tendon Organs1/1 -> LL Delay6/1
  LL Delay5/1 -> SDelay43/1
  SDelay43/1 -> L Swing Phase (coronal)/2(R_a_tgt)
  Sum3/1 -> LL Delay5/1
  SDelay44/1 -> L Swing Phase (coronal)/3(LceHAD)
  SDelay45/1 -> L Swing Phase (coronal)/4(LceHAB)
  MDelay22/1 -> "L Stance, Swing, Trans (coronal)"/2(Stance)
  MDelay17/1 -> "L Stance, Swing, Trans (coronal)"/3(CStance)
  SDelay46/1 -> [LStimHAB]
  SDelay40/1 -> [LStimHAD]
  "L Stance, Swing, Trans (coronal)"/1(S) -> Saturation3/1
  [LhipR_tgt] -> Sum3/2
  [thetaR] -> L GLU Golgi Tendon Organs2/1
  L GLU Golgi Tendon Organs2/1 -> Sum3/1
  [thetaR] -> Mux5/1
  [dthetaR] -> Mux5/2
  L Stance Phase (coronal)/2(S_M1 [HAB]) -> "L Stance, Swing, Trans (coronal)"/8(S_M1)
  [LFmHAB] -> SDelay39/1
  SDelay39/1 -> L Stance Phase (coronal)/5(FmHAB)
  SDelay35/1 -> [RStimHAB]
  SDelay37/1 -> [RStimHAD]
  L Stance Phase (sagittal)/7(S_M11 [SOL TA GAS]) -> "L Stance, Swing, Trans (sagittal)"/21(S_M11)
  [front_dv_L] -> Selector/1
  L Stance Phase (sagittal)1/7(S_M11 [SOL TA GAS]) -> "L Stance, Swing, Trans (sagittal)1"/21(S_M11)
  Selector/1 -> LL Delay9/1
  [front_dv_R] -> Selector1/1
  Selector1/1 -> LL Delay10/1
  LL Delay9/1 -> SDelay50/1
  SDelay50/1 -> L Stance Phase (sagittal)/12(COMVel)
  LL Delay10/1 -> SDelay51/1
  SDelay51/1 -> L Stance Phase (sagittal)1/12(COMVel)

== system nmc/NMC Model/etc ==
  note: Control Parameters
  Clock : Clock
  Constant{1,7,13..18,20,22} (10 alike) : Constant  Value=CtrlPar_VelocityFile_List
  Constant10 : Constant  Value=CtrlPar_Tr_List
  Constant11 : Constant  Value=CtrlPar_Tr_R_List
  Constant12 : Constant  Value=CtrlPar_theta0_List
  Constant2 : Constant  Value=CtrlPar_LL_List
  Constant3 : Constant  Value=CtrlPar_St_R_List
  Constant4 : Constant  Value=CtrlPar_FP_R_List
  Constant5 : Constant  Value=CtrlPar_St_List
  Constant6 : Constant  Value=CtrlPar_FP_List
  Constant8 : Constant  Value=CtrlPar_Sw_R_List
  Constant9 : Constant  Value=CtrlPar_Sw_List
  ParamScaling{,1..9} (10 alike) : nmc/ParamScaling
  To Current Workspace2 : ToWorkspace  VariableName=simout_tEnd  SaveFormat=Structure  SampleTime=-1
      settings: MaxDataPoints=1
  tag scope: FPCtrlPar=global, LLCtrlPar=global, R_FPCtrlPar=global, R_StCtrlPar=global, R_SwCtrlPar=global, R_TrCtrlPar=global, StCtrlPar=global, SwCtrlPar=global, TrCtrlPar=global, theta0=global
  wires:
  Constant17/1 -> ParamScaling9/2
  [NMC_CurVelocity] -> ParamScaling9/3
  ParamScaling9/1 -> [R_StCtrlPar]
  Constant3/1 -> ParamScaling9/1
  Constant15/1 -> ParamScaling8/2
  [NMC_CurVelocity] -> ParamScaling8/3
  ParamScaling8/1 -> [TrCtrlPar]
  Constant10/1 -> ParamScaling8/1
  Constant7/1 -> ParamScaling7/2
  [NMC_CurVelocity] -> ParamScaling7/3
  ParamScaling7/1 -> [SwCtrlPar]
  Constant9/1 -> ParamScaling7/1
  Constant22/1 -> ParamScaling6/2
  [NMC_CurVelocity] -> ParamScaling6/3
  ParamScaling6/1 -> [StCtrlPar]
  Constant5/1 -> ParamScaling6/1
  Constant20/1 -> ParamScaling5/2
  [NMC_CurVelocity] -> ParamScaling5/3
  ParamScaling5/1 -> [LLCtrlPar]
  Constant2/1 -> ParamScaling5/1
  Constant18/1 -> ParamScaling4/2
  [NMC_CurVelocity] -> ParamScaling4/3
  ParamScaling4/1 -> [FPCtrlPar]
  Constant6/1 -> ParamScaling4/1
  Constant16/1 -> ParamScaling3/2
  [NMC_CurVelocity] -> ParamScaling3/3
  ParamScaling3/1 -> [theta0]
  Constant12/1 -> ParamScaling3/1
  Constant14/1 -> ParamScaling2/2
  [NMC_CurVelocity] -> ParamScaling2/3
  ParamScaling2/1 -> [R_TrCtrlPar]
  Constant11/1 -> ParamScaling2/1
  Constant1/1 -> ParamScaling1/2
  [NMC_CurVelocity] -> ParamScaling1/3
  ParamScaling1/1 -> [R_SwCtrlPar]
  Constant8/1 -> ParamScaling1/1
  Constant13/1 -> ParamScaling/2
  [NMC_CurVelocity] -> ParamScaling/3
  ParamScaling/1 -> [R_FPCtrlPar]
  Constant4/1 -> ParamScaling/1
  Clock/1 -> To Current Workspace2/1

== system nmc/LopesToGeyer_angles/AnklePredictorLeft/LeftStance ==
  MeasPhase : Inport
  Clock : Clock
      settings: Decimation=1E6
  Constant : Constant  Value=MeanStepsAnkle
  "Frequency " : Stateflow chart  TreatAsAtomicUnit=on
  "mean_freq " : Outport
  count : Outport  Port=2
  wires:
  "Frequency "/1(count) -> count/1
  "Frequency "/2(mean_freq) -> "mean_freq "/1
  Clock/1 -> "Frequency "/1(time_sig)
  MeasPhase/1 -> "Frequency "/2(InSig)
  Constant/1 -> "Frequency "/3(N)

== system nmc/LopesToGeyer_angles/AnklePredictorLeft/LeftStance1 ==
  MeasPhase : Inport
  Clock : Clock
      settings: Decimation=1E6
  Constant : Constant  Value=MeanStepsAnkle
  "Frequency " : Stateflow chart  TreatAsAtomicUnit=on
  "mean_freq " : Outport
  count : Outport  Port=2
  wires:
  Constant/1 -> "Frequency "/3(N)
  MeasPhase/1 -> "Frequency "/2(InSig)
  Clock/1 -> "Frequency "/1(time_sig)
  "Frequency "/2(mean_freq) -> "mean_freq "/1
  "Frequency "/1(count) -> count/1

== system nmc/LopesToGeyer_angles/AnklePredictorLeft/MeanReady? ==
  Compare To Constant2 : simulink/Logic and Bit Operations/Compare To Constant  relop=>  const=MeanStepsAnkle  OutDataTypeStr=boolean
  Compare To Constant3 : simulink/Logic and Bit Operations/Compare To Constant  relop=>  const=MeanStepsAnkle  OutDataTypeStr=boolean
  Logical Operator : Logic  AllPortsSameDT=off  OutDataTypeStr=boolean
  "Ready " : Outport
  wires:
  [CountStanceL] -> Compare To Constant2/1
  Compare To Constant2/1 -> Logical Operator/2
  Compare To Constant3/1 -> Logical Operator/1
  [CountSwingL] -> Compare To Constant3/1
  Logical Operator/1 -> "Ready "/1

== system nmc/LopesToGeyer_angles/AnklePredictorLeft/Shape estimator left ==
  Cur_phase : Inport
  mean_freq_swing : Inport  Port=2
  mean_freq_stance : Inport  Port=3
  Enable : EnablePort  StatesWhenEnabling=reset  ZeroCross=off
  Compare To Constant : simulink/Logic and Bit Operations/Compare To Constant  relop===  const=0  OutDataTypeStr=boolean
  Compare To Constant1 : simulink/Logic and Bit Operations/Compare To Constant  relop===  const=1  OutDataTypeStr=boolean
  Cur_phase1 : InportShadow
  Phase 1 : Subsystem
  Phase 2 : Subsystem
  Switch : Switch  Criteria=u2 ~= 0
  Shape : Outport  OutputWhenDisabled=reset  InitialOutput=0
  wires:
  Cur_phase/1 -> Compare To Constant/1, Compare To Constant1/1
  Switch/1 -> Shape/1
  Phase 2/1(Shape_output) -> Switch/1
  Phase 1/1(Shape_output) -> Switch/3
  Cur_phase1/1 -> Switch/2
  Compare To Constant/1 -> Phase 1/Enable
  Compare To Constant1/1 -> Phase 2/Enable
  mean_freq_swing/1 -> Phase 1/1(mean_freq)
  mean_freq_stance/1 -> Phase 2/1(mean_freq)

== system nmc/LopesToGeyer_angles/AnklePredictorRight/LeftStance ==
  MeasPhase : Inport
  Clock : Clock
      settings: Decimation=1E6
  Constant : Constant  Value=MeanStepsAnkle
  "Frequency " : Stateflow chart  TreatAsAtomicUnit=on
  "mean_freq " : Outport
  count : Outport  Port=2
  wires:
  Constant/1 -> "Frequency "/3(N)
  MeasPhase/1 -> "Frequency "/2(InSig)
  Clock/1 -> "Frequency "/1(time_sig)
  "Frequency "/2(mean_freq) -> "mean_freq "/1
  "Frequency "/1(count) -> count/1
